simulink model "Australian14gen_inertia"  (R2017b)
settings: Solver=ode23tb  StartTime=0.0  StopTime=50  FixedStep=1e-3  RelTol=1e-3  AbsTol=1e-3  EnableMultiTasking=on
PreLoadFcn:
  | dataaustralian14gen
values from neighbouring files (symbols this model uses):
  alpha = -sys.follin.opt.alpha*1e8    [main_following.m]    (also in optimgains.mat = [-2447350365.29 -12566370614.4 -12566370614.4 -11730281347.7)
  bus_v = [ 101	15 ... (first row only)    [dataaustralian14gen.m]
  comp = [ 1	211	0	0 ... (first row only)    [dataaustralian14gen.m]
  dist = sys.follin.dist    [main_following.m]    (also in main_forming.m = sys.formin.dist)
  Exc = [ 101	0	 200	0.1	    13.25  2.5	 0	0       0       0       0       0 ... (first row only)    [dataaustralian14gen.m]
  FH = 13    [dataaustralian14gen.m]
  FI = 1    [dataaustralian14gen.m]
  FL = .1    (= 0.1)    [dataaustralian14gen.m]
  G_data = [ 101	333.3	15	3.6	0.14	1.1	0.65	0.25	8.5     0.25	0.05	0       0       0.25	0.2 	0 ... (first row only)    [dataaustralian14gen.m]
  KH = 120    [dataaustralian14gen.m]
  KI = 10    [dataaustralian14gen.m]
  KL = 10    [dataaustralian14gen.m]
  Kvsc = [-4.89904313526 -21.043852985 -7.4754770322 -20.8245159401 -7.65455531538 -20.65157337 -7.20128124012 -20.8334958357 -6.74777960012 -20.6206111903 -7.78863485578 -20.7555924998 ... (30 elements, 2x15)]    [optimgains.mat]
  line = [ 102	217	0.0084	0.0667	0.817	330	1 ... (first row only)    [dataaustralian14gen.m]
  load_mag = load_case4    [dataaustralian14gen.m]
  p = p_case4    [dataaustralian14gen.m]
  Pinit = zeros(15,1)    [dataaustralian14gen.m]
  PLL_Ki = 2/500    (= 0.004)    [dataaustralian14gen.m]
  PLL_Kp = 2/500    (= 0.004)    [dataaustralian14gen.m]
  PSSMODEL = 1    [dataaustralian14gen.m]
  trans = [ 1	101	102	15	330	333.3	12	12 ... (first row only)    [dataaustralian14gen.m]
undefined symbols (not defined in the file or in its folder): D1, Delta, sys, thetavsc0, Vbase
libraries: powerlib x388, Library x60, powerlib_meascontrol x15, sps_avr x10, powerlib_extras x4
(part 4 of 5)

== system Australian14gen_inertia/VI215_form ==
  Complex to Magnitude-Angle : ComplexToMagnitudeAngle
  Complex to Magnitude-Angle1 : ComplexToMagnitudeAngle
  Demux : Demux  Outputs=[3 3]
  Filter215 : Library/Filter  r=r_fil  l=l_fil  c=c_fil
  Gain : Gain  Gain=[1 0 0]  Multiplication=Matrix(K*u) (u vector)
  Gain1 : Gain  Gain=[1 0 0]  Multiplication=Matrix(K*u) (u vector)
  INV215 : Library/INV  fn=50  Ub=Vbase(4)  Pref=Pinit(4)  ang=thetavsc0(4)  K2=Kvsc(1,4)  K1=Kvsc(2,4)
  Load Flow Bus26 : powerlib/Measurements/Load Flow Bus  Commented=on  LConnTagsString=a  Phases=single  Connectors=on one side  ID=B215_vsw  Vbase=20e3  Vref=1  Vangle=0  VLF=1  VLFb=1  VLFc=1  angleLF=23.87  angleLFb=0  angleLFc=0
      settings: AttributesFormatString=%<ID>\n%<Vbase>V\n%<VLF>pu\n%<angleLF>deg.  SourceProductName=Simscape Power Systems
  Mux : Mux  Inputs=2
  Mux1 : Mux  Inputs=2
  Mux29 : Mux  Inputs=3
  Scope : Scope
  Scope1 : Scope  NumInputPorts=2
  Sum : Sum  Inputs=|+-
  fake_VSC_215 : powerlib/Electrical Sources/Three-Phase Source  Commented=on  InternalConnection=Yg  VoltagePhases=off  Voltage=(20000)*1  PhaseAngle=23.8703  Voltage_phases=[25e3 25e3 25e3]/sqrt(3)  PhaseAngles_phases=[0 -120 +120]  Frequency=50  NonIdealSource=off  SpecifyImpedance=off  Resistance=0  Inductance=0  ShortCircuitLevel=100e6  BaseVoltage=20e3  XRratio=7  BusType=PV  Pref=0  Qref=0  Prefabc=[10e3, 10e3, 10e3]  Qrefabc=[0, 0, 0]  Qmin=-inf  Qmax=inf
  u215 : Constant  Value=0
  A : PMIOPort  Port=1  Side=Left
  B : PMIOPort  Port=2  Side=Left
  C : PMIOPort  Port=3  Side=Left
  tag scope: P215=global, Q215=global, w215=global
  wires:
  u215/1 -> INV215/1
  INV215/3 -> Mux29/2
  INV215/2 -> Mux29/1
  Filter215/2 -> [Q215]
  INV215/1 -> [P215]
  INV215/4 -> Mux29/3
  Mux29/1 -> [w215]
  Filter215/1 -> INV215/2
  Mux/1 -> Scope1/1
  Sum/1 -> Scope/1
  Complex to Magnitude-Angle1/2 -> Mux1/2
  Gain/1 -> Complex to Magnitude-Angle/1
  Complex to Magnitude-Angle/1 -> Mux/1
  Demux/2 -> Gain1/1, Sum/2
  Filter215/3 -> Demux/1
  Demux/1 -> Gain/1, Sum/1
  Complex to Magnitude-Angle/2 -> Mux1/1
  Gain1/1 -> Complex to Magnitude-Angle1/1
  Mux1/1 -> Scope1/2
  Complex to Magnitude-Angle1/1 -> Mux/2
  connections:
  Filter215/LConn1 -- INV215/LConn1 -- Load Flow Bus26/LConn1 -- fake_VSC_215/RConn1
  Filter215/LConn2 -- INV215/LConn2 -- fake_VSC_215/RConn2
  Filter215/LConn3 -- INV215/LConn3 -- fake_VSC_215/RConn3
  C/RConn1 -- Filter215/RConn3
  Filter215/RConn2 -- B/RConn1
  A/RConn1 -- Filter215/RConn1

== system Australian14gen_inertia/VI216 ==
  Constant : Constant  Value=0
  Gain : Gain  Gain=-1
  Gain1 : Gain  Gain=[0 1]  Multiplication=Matrix(K*u) (u vector)
  Mux : Mux  Inputs=2
  Mux1 : Mux  Inputs=3
  PLL : Library/PLL  Kp=PLL_Kp  Ki=PLL_Ki  tau=PLL_tau  theta0=14.521  omega0=0
  "Power (3ph, Phasor)" : powerlib_meascontrol/Measurements/Power (3ph, Phasor)
      settings: SourceProductName=Simscape Power Systems  SourceProductBaseCode=PS
  Three-Phase V-I Measurement : powerlib/Measurements/Three-Phase V-I Measurement  VoltageMeasurement=phase-to-ground  SetLabelV=off  LabelV=Vabc  Vpu=off  VpuLL=off  CurrentMeasurement=yes  SetLabelI=off  LabelI=Iabc  Ipu=off  Pbase=100e6  Vbase=500e3  OutputType=Complex  PhasorSimulation=on  PSBequivalent=0
  dP102_vi : Library/dP102_vi  d=alpha(5)  m=alpha(20)
  virtin : powerlib/Elements/Three-Phase Dynamic Load  NominalVoltage=[20e3 50 ]  ActiveReactivePowers=[0 0]  PositiveSequence=[1.0263 14.521]  ExternalControl=on  NpNq="[0  0]"  TimeConstants="[0  0  0  0]"  MinimumVoltage=0.01  Tfilter=1e-1  LoadFlowParameters=[4 50000000 0 0 25000000]
      settings: SourceProductName=Simscape Power Systems  SourceProductBaseCode=PS
  A : PMIOPort  Port=1  Side=Right
  B : PMIOPort  Port=2  Side=Right
  C : PMIOPort  Port=3  Side=Right
  tag scope: P216=global, Q216=global, w216=global
  wires:
  Mux/1 -> Gain/1
  Gain/1 -> virtin/1
  Constant/1 -> Mux/2
  dP102_vi/1 -> Mux/1
  [Vabc_B216_vi] -> PLL/1
  PLL/1 -> Mux1/1, dP102_vi/1
  Mux1/1 -> [w216]
  PLL/2 -> Mux1/2, dP102_vi/2
  "Power (3ph, Phasor)"/1 -> [P216]
  Three-Phase V-I Measurement/1 -> "Power (3ph, Phasor)"/1
  "Power (3ph, Phasor)"/2 -> [Q216]
  Three-Phase V-I Measurement/2 -> "Power (3ph, Phasor)"/2
  PLL/3 -> Gain1/1
  Gain1/1 -> Mux1/3
  connections:
  C/RConn1 -- Three-Phase V-I Measurement/RConn3
  B/RConn1 -- Three-Phase V-I Measurement/RConn2
  A/RConn1 -- Three-Phase V-I Measurement/RConn1
  virtin/LConn3 -- Three-Phase V-I Measurement/LConn3
  virtin/LConn2 -- Three-Phase V-I Measurement/LConn2
  virtin/LConn1 -- Three-Phase V-I Measurement/LConn1

== system Australian14gen_inertia/VI216_form ==
  Complex to Magnitude-Angle : ComplexToMagnitudeAngle
  Complex to Magnitude-Angle1 : ComplexToMagnitudeAngle
  Demux : Demux  Outputs=[3 3]
  Filter216 : Library/Filter  r=r_fil  l=l_fil  c=c_fil
  Gain : Gain  Gain=[1 0 0]  Multiplication=Matrix(K*u) (u vector)
  Gain1 : Gain  Gain=[1 0 0]  Multiplication=Matrix(K*u) (u vector)
  INV216 : Library/INV  fn=50  Ub=Vbase(5)  Pref=Pinit(5)  ang=thetavsc0(5)  K2=Kvsc(1,5)  K1=Kvsc(2,5)
  Load Flow Bus25 : powerlib/Measurements/Load Flow Bus  Commented=on  LConnTagsString=a  Phases=single  Connectors=on one side  ID=B216_vsw  Vbase=20e3  Vref=1  Vangle=0  VLF=1  VLFb=1  VLFc=1  angleLF=14.02  angleLFb=0  angleLFc=0
      settings: AttributesFormatString=%<ID>\n%<Vbase>V\n%<VLF>pu\n%<angleLF>deg.  SourceProductName=Simscape Power Systems
  Mux : Mux  Inputs=2
  Mux1 : Mux  Inputs=2
  Mux23 : Mux  Inputs=3
  Scope : Scope
  Scope1 : Scope  NumInputPorts=2
  Sum : Sum  Inputs=|+-
  fake_VSC_216 : powerlib/Electrical Sources/Three-Phase Source  Commented=on  InternalConnection=Yg  VoltagePhases=off  Voltage=(20000)*1  PhaseAngle=14.0249  Voltage_phases=[25e3 25e3 25e3]/sqrt(3)  PhaseAngles_phases=[0 -120 +120]  Frequency=50  NonIdealSource=off  SpecifyImpedance=off  Resistance=0  Inductance=0  ShortCircuitLevel=100e6  BaseVoltage=20e3  XRratio=7  BusType=PV  Pref=0  Qref=0  Prefabc=[10e3, 10e3, 10e3]  Qrefabc=[0, 0, 0]  Qmin=-inf  Qmax=inf
  u216 : Constant  Value=0
  A : PMIOPort  Port=1  Side=Left
  B : PMIOPort  Port=2  Side=Left
  C : PMIOPort  Port=3  Side=Left
  tag scope: P216=global, Q216=global, w216=global
  wires:
  INV216/3 -> Mux23/2
  Filter216/1 -> INV216/2
  u216/1 -> INV216/1
  INV216/4 -> Mux23/3
  Mux23/1 -> [w216]
  INV216/1 -> [P216]
  INV216/2 -> Mux23/1
  Filter216/2 -> [Q216]
  Mux/1 -> Scope1/1
  Sum/1 -> Scope/1
  Complex to Magnitude-Angle1/2 -> Mux1/2
  Gain/1 -> Complex to Magnitude-Angle/1
  Complex to Magnitude-Angle/1 -> Mux/1
  Demux/2 -> Gain1/1, Sum/2
  Filter216/3 -> Demux/1
  Demux/1 -> Gain/1, Sum/1
  Complex to Magnitude-Angle/2 -> Mux1/1
  Gain1/1 -> Complex to Magnitude-Angle1/1
  Mux1/1 -> Scope1/2
  Complex to Magnitude-Angle1/1 -> Mux/2
  connections:
  INV216/LConn3 -- Filter216/LConn3 -- fake_VSC_216/RConn3
  INV216/LConn2 -- Filter216/LConn2 -- fake_VSC_216/RConn2
  Load Flow Bus25/LConn1 -- Filter216/LConn1 -- fake_VSC_216/RConn1 -- INV216/LConn1
  Filter216/RConn1 -- A/RConn1
  Filter216/RConn2 -- B/RConn1
  Filter216/RConn3 -- C/RConn1

== system Australian14gen_inertia/VI308 ==
  Constant : Constant  Value=0
  Gain : Gain  Gain=-1
  Gain1 : Gain  Gain=[0 1]  Multiplication=Matrix(K*u) (u vector)
  Mux : Mux  Inputs=2
  Mux1 : Mux  Inputs=3
  PLL : Library/PLL  Kp=PLL_Kp  Ki=PLL_Ki  tau=PLL_tau  theta0=-6.09646  omega0=0
  "Power (3ph, Phasor)" : powerlib_meascontrol/Measurements/Power (3ph, Phasor)
      settings: SourceProductName=Simscape Power Systems  SourceProductBaseCode=PS
  Three-Phase V-I Measurement : powerlib/Measurements/Three-Phase V-I Measurement  VoltageMeasurement=phase-to-ground  SetLabelV=off  LabelV=Vabc  Vpu=off  VpuLL=off  CurrentMeasurement=yes  SetLabelI=off  LabelI=Iabc  Ipu=off  Pbase=100e6  Vbase=500e3  OutputType=Complex  PhasorSimulation=on  PSBequivalent=0
  dP102_vi : Library/dP102_vi  d=alpha(6)  m=alpha(21)
  virtin : powerlib/Elements/Three-Phase Dynamic Load  NominalVoltage=[ 20e3 50 ]  ActiveReactivePowers=[0 0]  PositiveSequence=[1.0559 -6.09646]  ExternalControl=on  NpNq="[0  0]"  TimeConstants="[0  0  0  0]"  MinimumVoltage=0.01  Tfilter=1e-1  LoadFlowParameters=[4 50000000 0 0 25000000]
      settings: SourceProductName=Simscape Power Systems  SourceProductBaseCode=PS
  A : PMIOPort  Port=1  Side=Right
  B : PMIOPort  Port=2  Side=Right
  C : PMIOPort  Port=3  Side=Right
  tag scope: P308=global, Q308=global, w308=global
  wires:
  Mux/1 -> Gain/1
  Gain/1 -> virtin/1
  Constant/1 -> Mux/2
  dP102_vi/1 -> Mux/1
  [Vabc_B308_vi] -> PLL/1
  PLL/1 -> Mux1/1, dP102_vi/1
  Mux1/1 -> [w308]
  PLL/2 -> dP102_vi/2, Mux1/2
  "Power (3ph, Phasor)"/1 -> [P308]
  Three-Phase V-I Measurement/1 -> "Power (3ph, Phasor)"/1
  "Power (3ph, Phasor)"/2 -> [Q308]
  Three-Phase V-I Measurement/2 -> "Power (3ph, Phasor)"/2
  PLL/3 -> Gain1/1
  Gain1/1 -> Mux1/3
  connections:
  virtin/LConn1 -- Three-Phase V-I Measurement/LConn1
  C/RConn1 -- Three-Phase V-I Measurement/RConn3
  virtin/LConn3 -- Three-Phase V-I Measurement/LConn3
  B/RConn1 -- Three-Phase V-I Measurement/RConn2
  virtin/LConn2 -- Three-Phase V-I Measurement/LConn2
  A/RConn1 -- Three-Phase V-I Measurement/RConn1

== system Australian14gen_inertia/VI308_form ==
  Complex to Magnitude-Angle : ComplexToMagnitudeAngle
  Complex to Magnitude-Angle1 : ComplexToMagnitudeAngle
  Demux : Demux  Outputs=[3 3]
  Filter308 : Library/Filter  r=r_fil  l=l_fil  c=c_fil
  Gain : Gain  Gain=[1 0 0]  Multiplication=Matrix(K*u) (u vector)
  Gain1 : Gain  Gain=[1 0 0]  Multiplication=Matrix(K*u) (u vector)
  INV308 : Library/INV  fn=50  Ub=Vbase(6)  Pref=Pinit(6)  ang=thetavsc0(6)  K2=Kvsc(1,6)  K1=Kvsc(2,6)
  Load Flow Bus20 : powerlib/Measurements/Load Flow Bus  Commented=on  LConnTagsString=a  Phases=single  Connectors=on one side  ID=B308_vsw  Vbase=20e3  Vref=1  Vangle=0  VLF=1  VLFb=1  VLFc=1  angleLF=-6.338  angleLFb=0  angleLFc=0
      settings: AttributesFormatString=%<ID>\n%<Vbase>V\n%<VLF>pu\n%<angleLF>deg.  SourceProductName=Simscape Power Systems
  Mux : Mux  Inputs=2
  Mux1 : Mux  Inputs=2
  Mux19 : Mux  Inputs=3
  Scope : Scope
  Scope1 : Scope  NumInputPorts=2
  Sum : Sum  Inputs=|+-
  fake_VSC_308 : powerlib/Electrical Sources/Three-Phase Source  Commented=on  InternalConnection=Yg  VoltagePhases=off  Voltage=(20000)*1  PhaseAngle=-6.3379  Voltage_phases=[25e3 25e3 25e3]/sqrt(3)  PhaseAngles_phases=[0 -120 +120]  Frequency=50  NonIdealSource=off  SpecifyImpedance=off  Resistance=0  Inductance=0  ShortCircuitLevel=100e6  BaseVoltage=20e3  XRratio=7  BusType=PV  Pref=0  Qref=0  Prefabc=[10e3, 10e3, 10e3]  Qrefabc=[0, 0, 0]  Qmin=-inf  Qmax=inf
  u308 : Constant  Value=0
  A : PMIOPort  Port=1  Side=Left
  B : PMIOPort  Port=2  Side=Left
  C : PMIOPort  Port=3  Side=Left
  tag scope: P308=global, Q308=global, w308=global
  wires:
  INV308/4 -> Mux19/3
  Mux19/1 -> [w308]
  u308/1 -> INV308/1
  INV308/2 -> Mux19/1
  INV308/3 -> Mux19/2
  INV308/1 -> [P308]
  Filter308/1 -> INV308/2
  Filter308/2 -> [Q308]
  Mux/1 -> Scope1/1
  Sum/1 -> Scope/1
  Complex to Magnitude-Angle1/2 -> Mux1/2
  Gain/1 -> Complex to Magnitude-Angle/1
  Complex to Magnitude-Angle/1 -> Mux/1
  Demux/2 -> Gain1/1, Sum/2
  Filter308/3 -> Demux/1
  Demux/1 -> Gain/1, Sum/1
  Complex to Magnitude-Angle/2 -> Mux1/1
  Gain1/1 -> Complex to Magnitude-Angle1/1
  Mux1/1 -> Scope1/2
  Complex to Magnitude-Angle1/1 -> Mux/2
  connections:
  INV308/LConn3 -- Load Flow Bus20/LConn1 -- Filter308/LConn3 -- fake_VSC_308/RConn3
  INV308/LConn1 -- fake_VSC_308/RConn1 -- Filter308/LConn1
  INV308/LConn2 -- fake_VSC_308/RConn2 -- Filter308/LConn2
  B/RConn1 -- Filter308/RConn2
  C/RConn1 -- Filter308/RConn3
  A/RConn1 -- Filter308/RConn1

== system Australian14gen_inertia/VI309 ==
  Constant : Constant  Value=0
  Gain : Gain  Gain=-1
  Gain1 : Gain  Gain=[0 1]  Multiplication=Matrix(K*u) (u vector)
  Mux : Mux  Inputs=2
  Mux1 : Mux  Inputs=3
  PLL : Library/PLL  Kp=PLL_Kp  Ki=PLL_Ki  tau=PLL_tau  theta0=126.6523  omega0=0
  "Power (3ph, Phasor)" : powerlib_meascontrol/Measurements/Power (3ph, Phasor)
      settings: SourceProductName=Simscape Power Systems  SourceProductBaseCode=PS
  Three-Phase V-I Measurement : powerlib/Measurements/Three-Phase V-I Measurement  VoltageMeasurement=phase-to-ground  SetLabelV=off  LabelV=Vabc  Vpu=off  VpuLL=off  CurrentMeasurement=yes  SetLabelI=off  LabelI=Iabc  Ipu=off  Pbase=100e6  Vbase=500e3  OutputType=Complex  PhasorSimulation=on  PSBequivalent=0
  dP102_vi : Library/dP102_vi  d=alpha(7)  m=alpha(22)
  virtin : powerlib/Elements/Three-Phase Dynamic Load  NominalVoltage=[ 15e3 50 ]  ActiveReactivePowers=[0 0]  PositiveSequence=[1.04736 5.11816]  ExternalControl=on  NpNq="[0  0]"  TimeConstants="[0  0  0  0]"  MinimumVoltage=0.01  Tfilter=1e-1  LoadFlowParameters=[4 50000000 0 0 25000000]
      settings: SourceProductName=Simscape Power Systems  SourceProductBaseCode=PS
  A : PMIOPort  Port=1  Side=Right
  B : PMIOPort  Port=2  Side=Right
  C : PMIOPort  Port=3  Side=Right
  tag scope: P309=global, Q309=global, w309=global
  wires:
  Mux/1 -> Gain/1
  Gain/1 -> virtin/1
  Constant/1 -> Mux/2
  dP102_vi/1 -> Mux/1
  [Vabc_B309_vi] -> PLL/1
  PLL/1 -> Mux1/1, dP102_vi/1
  Mux1/1 -> [w309]
  PLL/2 -> Mux1/2, dP102_vi/2
  "Power (3ph, Phasor)"/1 -> [P309]
  Three-Phase V-I Measurement/1 -> "Power (3ph, Phasor)"/1
  "Power (3ph, Phasor)"/2 -> [Q309]
  Three-Phase V-I Measurement/2 -> "Power (3ph, Phasor)"/2
  PLL/3 -> Gain1/1
  Gain1/1 -> Mux1/3
  connections:
  virtin/LConn1 -- Three-Phase V-I Measurement/LConn1
  C/RConn1 -- Three-Phase V-I Measurement/RConn3
  virtin/LConn3 -- Three-Phase V-I Measurement/LConn3
  B/RConn1 -- Three-Phase V-I Measurement/RConn2
  virtin/LConn2 -- Three-Phase V-I Measurement/LConn2
  A/RConn1 -- Three-Phase V-I Measurement/RConn1

== system Australian14gen_inertia/VI309_form ==
  Complex to Magnitude-Angle : ComplexToMagnitudeAngle
  Complex to Magnitude-Angle1 : ComplexToMagnitudeAngle
  Demux : Demux  Outputs=[3 3]
  Filter309 : Library/Filter  r=r_fil  l=l_fil  c=c_fil
  Gain : Gain  Gain=[1 0 0]  Multiplication=Matrix(K*u) (u vector)
  Gain1 : Gain  Gain=[1 0 0]  Multiplication=Matrix(K*u) (u vector)
  INV309 : Library/INV  fn=50  Ub=Vbase(7)  Pref=Pinit(7)  ang=thetavsc0(7)  K2=Kvsc(1,7)  K1=Kvsc(2,7)
  Load Flow Bus23 : powerlib/Measurements/Load Flow Bus  Commented=on  LConnTagsString=a  Phases=single  Connectors=on one side  ID=B309_vsw  Vbase=15e3  Vref=1  Vangle=0  VLF=1  VLFb=1  VLFc=1  angleLF=4.793  angleLFb=0  angleLFc=0
      settings: AttributesFormatString=%<ID>\n%<Vbase>V\n%<VLF>pu\n%<angleLF>deg.  SourceProductName=Simscape Power Systems
  Mux : Mux  Inputs=2
  Mux1 : Mux  Inputs=2
  Mux28 : Mux  Inputs=3
  Scope : Scope
  Scope1 : Scope  NumInputPorts=2
  Sum : Sum  Inputs=|+-
  fake_VSC_309 : powerlib/Electrical Sources/Three-Phase Source  Commented=on  InternalConnection=Yg  VoltagePhases=off  Voltage=(15000)*1  PhaseAngle=4.7928  Voltage_phases=[25e3 25e3 25e3]/sqrt(3)  PhaseAngles_phases=[0 -120 +120]  Frequency=50  NonIdealSource=off  SpecifyImpedance=off  Resistance=0  Inductance=0  ShortCircuitLevel=100e6  BaseVoltage=20e3  XRratio=7  BusType=PV  Pref=0  Qref=0  Prefabc=[10e3, 10e3, 10e3]  Qrefabc=[0, 0, 0]  Qmin=-inf  Qmax=inf
  u309 : Constant  Value=0
  A : PMIOPort  Port=1  Side=Right
  B : PMIOPort  Port=2  Side=Right
  C : PMIOPort  Port=3  Side=Right
  tag scope: P309=global, Q309=global, w309=global
  wires:
  INV309/1 -> [P309]
  Filter309/1 -> INV309/2
  INV309/3 -> Mux28/2
  Mux28/1 -> [w309]
  INV309/2 -> Mux28/1
  Filter309/2 -> [Q309]
  u309/1 -> INV309/1
  INV309/4 -> Mux28/3
  Mux/1 -> Scope1/1
  Sum/1 -> Scope/1
  Complex to Magnitude-Angle1/2 -> Mux1/2
  Gain/1 -> Complex to Magnitude-Angle/1
  Complex to Magnitude-Angle/1 -> Mux/1
  Demux/2 -> Gain1/1, Sum/2
  Filter309/3 -> Demux/1
  Demux/1 -> Gain/1, Sum/1
  Complex to Magnitude-Angle/2 -> Mux1/1
  Gain1/1 -> Complex to Magnitude-Angle1/1
  Mux1/1 -> Scope1/2
  Complex to Magnitude-Angle1/1 -> Mux/2
  connections:
  INV309/LConn3 -- fake_VSC_309/RConn3 -- Filter309/LConn3
  INV309/LConn1 -- Load Flow Bus23/LConn1 -- Filter309/LConn1 -- fake_VSC_309/RConn1
  INV309/LConn2 -- fake_VSC_309/RConn2 -- Filter309/LConn2
  A/RConn1 -- Filter309/RConn1
  B/RConn1 -- Filter309/RConn2
  C/RConn1 -- Filter309/RConn3

== system Australian14gen_inertia/VI312 ==
  Constant : Constant  Value=0
  Gain : Gain  Gain=-1
  Gain1 : Gain  Gain=[0 1]  Multiplication=Matrix(K*u) (u vector)
  Mux : Mux  Inputs=2
  Mux1 : Mux  Inputs=3
  PLL : Library/PLL  Kp=PLL_Kp  Ki=PLL_Ki  tau=PLL_tau  theta0=3.98868  omega0=0
  "Power (3ph, Phasor)" : powerlib_meascontrol/Measurements/Power (3ph, Phasor)
      settings: SourceProductName=Simscape Power Systems  SourceProductBaseCode=PS
  Three-Phase V-I Measurement : powerlib/Measurements/Three-Phase V-I Measurement  VoltageMeasurement=phase-to-ground  SetLabelV=off  LabelV=Vabc  Vpu=off  VpuLL=off  CurrentMeasurement=yes  SetLabelI=off  LabelI=Iabc  Ipu=off  Pbase=100e6  Vbase=500e3  OutputType=Complex  PhasorSimulation=on  PSBequivalent=0
  dP102_vi : Library/dP102_vi  d=alpha(8)  m=alpha(23)
  virtin : powerlib/Elements/Three-Phase Dynamic Load  NominalVoltage=[ 20e3 50 ]  ActiveReactivePowers=[0 0]  PositiveSequence=[0.998867 3.98868]  ExternalControl=on  NpNq="[0  0]"  TimeConstants="[0  0  0  0]"  MinimumVoltage=0.01  Tfilter=1e-1  LoadFlowParameters=[4 50000000 0 0 25000000]
      settings: SourceProductName=Simscape Power Systems  SourceProductBaseCode=PS
  A : PMIOPort  Port=1  Side=Right
  B : PMIOPort  Port=2  Side=Right
  C : PMIOPort  Port=3  Side=Right
  tag scope: P312=global, Q312=global, w312=global
  wires:
  Mux/1 -> Gain/1
  Gain/1 -> virtin/1
  Constant/1 -> Mux/2
  dP102_vi/1 -> Mux/1
  [Vabc_B312_vi] -> PLL/1
  PLL/1 -> Mux1/1, dP102_vi/1
  Mux1/1 -> [w312]
  PLL/2 -> Mux1/2, dP102_vi/2
  "Power (3ph, Phasor)"/1 -> [P312]
  Three-Phase V-I Measurement/1 -> "Power (3ph, Phasor)"/1
  "Power (3ph, Phasor)"/2 -> [Q312]
  Three-Phase V-I Measurement/2 -> "Power (3ph, Phasor)"/2
  PLL/3 -> Gain1/1
  Gain1/1 -> Mux1/3
  connections:
  virtin/LConn1 -- Three-Phase V-I Measurement/LConn1
  C/RConn1 -- Three-Phase V-I Measurement/RConn3
  virtin/LConn3 -- Three-Phase V-I Measurement/LConn3
  B/RConn1 -- Three-Phase V-I Measurement/RConn2
  virtin/LConn2 -- Three-Phase V-I Measurement/LConn2
  A/RConn1 -- Three-Phase V-I Measurement/RConn1

== system Australian14gen_inertia/VI312_form ==
  Complex to Magnitude-Angle : ComplexToMagnitudeAngle
  Complex to Magnitude-Angle1 : ComplexToMagnitudeAngle
  Demux : Demux  Outputs=[3 3]
  Filter312 : Library/Filter  r=r_fil  l=l_fil  c=c_fil
  Gain : Gain  Gain=[1 0 0]  Multiplication=Matrix(K*u) (u vector)
  Gain1 : Gain  Gain=[1 0 0]  Multiplication=Matrix(K*u) (u vector)
  INV312 : Library/INV  fn=50  Ub=Vbase(8)  Pref=Pinit(8)  ang=thetavsc0(8)  K2=Kvsc(1,8)  K1=Kvsc(2,8)
  Load Flow Bus22 : powerlib/Measurements/Load Flow Bus  Commented=on  LConnTagsString=a  Phases=single  Connectors=on one side  ID=B312_vsw  Vbase=20e3  Vref=1  Vangle=0  VLF=1  VLFb=1  VLFc=1  angleLF=3.684  angleLFb=0  angleLFc=0
      settings: AttributesFormatString=%<ID>\n%<Vbase>V\n%<VLF>pu\n%<angleLF>deg.  SourceProductName=Simscape Power Systems
  Mux : Mux  Inputs=2
  Mux1 : Mux  Inputs=2
  Mux17 : Mux  Inputs=3
  Scope : Scope
  Scope1 : Scope  NumInputPorts=2
  Sum : Sum  Inputs=|+-
  fake_VSC_312 : powerlib/Electrical Sources/Three-Phase Source  Commented=on  InternalConnection=Yg  VoltagePhases=off  Voltage=(20000)*1  PhaseAngle=3.6837  Voltage_phases=[25e3 25e3 25e3]/sqrt(3)  PhaseAngles_phases=[0 -120 +120]  Frequency=50  NonIdealSource=off  SpecifyImpedance=off  Resistance=0  Inductance=0  ShortCircuitLevel=100e6  BaseVoltage=20e3  XRratio=7  BusType=PV  Pref=0  Qref=0  Prefabc=[10e3, 10e3, 10e3]  Qrefabc=[0, 0, 0]  Qmin=-inf  Qmax=inf
  u312 : Constant  Value=0
  A : PMIOPort  Port=1  Side=Left
  B : PMIOPort  Port=2  Side=Left
  C : PMIOPort  Port=3  Side=Left
  tag scope: P312=global, Q312=global, w312=global
  wires:
  Filter312/2 -> [Q312]
  INV312/1 -> [P312]
  Filter312/1 -> INV312/2
  INV312/3 -> Mux17/2
  u312/1 -> INV312/1
  INV312/2 -> Mux17/1
  INV312/4 -> Mux17/3
  Mux17/1 -> [w312]
  Mux/1 -> Scope1/1
  Sum/1 -> Scope/1
  Complex to Magnitude-Angle1/2 -> Mux1/2
  Gain/1 -> Complex to Magnitude-Angle/1
  Complex to Magnitude-Angle/1 -> Mux/1
  Demux/2 -> Gain1/1, Sum/2
  Filter312/3 -> Demux/1
  Demux/1 -> Gain/1, Sum/1
  Complex to Magnitude-Angle/2 -> Mux1/1
  Gain1/1 -> Complex to Magnitude-Angle1/1
  Mux1/1 -> Scope1/2
  Complex to Magnitude-Angle1/1 -> Mux/2
  connections:
  INV312/LConn3 -- fake_VSC_312/RConn3 -- Filter312/LConn3
  INV312/LConn2 -- fake_VSC_312/RConn2 -- Filter312/LConn2
  INV312/LConn1 -- Load Flow Bus22/LConn1 -- fake_VSC_312/RConn1 -- Filter312/LConn1
  C/RConn1 -- Filter312/RConn3
  B/RConn1 -- Filter312/RConn2
  A/RConn1 -- Filter312/RConn1

== system Australian14gen_inertia/VI314 ==
  Constant : Constant  Value=0
  Gain : Gain  Gain=-1
  Gain1 : Gain  Gain=[0 1]  Multiplication=Matrix(K*u) (u vector)
  Mux : Mux  Inputs=2
  Mux1 : Mux  Inputs=3
  PLL : Library/PLL  Kp=PLL_Kp  Ki=PLL_Ki  tau=PLL_tau  theta0=-0.807945  omega0=0
  "Power (3ph, Phasor)" : powerlib_meascontrol/Measurements/Power (3ph, Phasor)
      settings: SourceProductName=Simscape Power Systems  SourceProductBaseCode=PS
  Three-Phase V-I Measurement : powerlib/Measurements/Three-Phase V-I Measurement  VoltageMeasurement=phase-to-ground  SetLabelV=off  LabelV=Vabc  Vpu=off  VpuLL=off  CurrentMeasurement=yes  SetLabelI=off  LabelI=Iabc  Ipu=off  Pbase=100e6  Vbase=500e3  OutputType=Complex  PhasorSimulation=on  PSBequivalent=0
  dP102_vi : Library/dP102_vi  d=alpha(9)  m=alpha(24)
  virtin : powerlib/Elements/Three-Phase Dynamic Load  NominalVoltage=[ 20e3 50 ]  ActiveReactivePowers=[0 0]  PositiveSequence=[0.999559 -0.807945]  ExternalControl=on  NpNq="[0  0]"  TimeConstants="[0  0  0  0]"  MinimumVoltage=0.01  Tfilter=1e-1  LoadFlowParameters=[4 50000000 0 0 25000000]
      settings: SourceProductName=Simscape Power Systems  SourceProductBaseCode=PS
  A : PMIOPort  Port=1  Side=Right
  B : PMIOPort  Port=2  Side=Right
  C : PMIOPort  Port=3  Side=Right
  tag scope: P314=global, Q314=global, w314=global
  wires:
  Mux/1 -> Gain/1
  Gain/1 -> virtin/1
  Constant/1 -> Mux/2
  dP102_vi/1 -> Mux/1
  [Vabc_B314_vi] -> PLL/1
  PLL/1 -> Mux1/1, dP102_vi/1
  Mux1/1 -> [w314]
  PLL/2 -> Mux1/2, dP102_vi/2
  "Power (3ph, Phasor)"/1 -> [P314]
  Three-Phase V-I Measurement/1 -> "Power (3ph, Phasor)"/1
  "Power (3ph, Phasor)"/2 -> [Q314]
  Three-Phase V-I Measurement/2 -> "Power (3ph, Phasor)"/2
  PLL/3 -> Gain1/1
  Gain1/1 -> Mux1/3
  connections:
  virtin/LConn1 -- Three-Phase V-I Measurement/LConn1
  C/RConn1 -- Three-Phase V-I Measurement/RConn3
  virtin/LConn3 -- Three-Phase V-I Measurement/LConn3
  B/RConn1 -- Three-Phase V-I Measurement/RConn2
  virtin/LConn2 -- Three-Phase V-I Measurement/LConn2
  A/RConn1 -- Three-Phase V-I Measurement/RConn1

== system Australian14gen_inertia/VI314_form ==
  Complex to Magnitude-Angle : ComplexToMagnitudeAngle
  Complex to Magnitude-Angle1 : ComplexToMagnitudeAngle
  Demux : Demux  Outputs=[3 3]
  Filter314 : Library/Filter  r=r_fil  l=l_fil  c=c_fil
  Gain : Gain  Gain=[1 0 0]  Multiplication=Matrix(K*u) (u vector)
  Gain1 : Gain  Gain=[1 0 0]  Multiplication=Matrix(K*u) (u vector)
  INV314 : Library/INV  fn=50  Ub=Vbase(9)  Pref=Pinit(9)  ang=thetavsc0(9)  K2=Kvsc(1,9)  K1=Kvsc(2,9)
  Load Flow Bus21 : powerlib/Measurements/Load Flow Bus  Commented=on  LConnTagsString=a  Phases=single  Connectors=on one side  ID=B314_vsw  Vbase=20e3  Vref=1  Vangle=0  VLF=1  VLFb=1  VLFc=1  angleLF=-1.099  angleLFb=0  angleLFc=0
      settings: AttributesFormatString=%<ID>\n%<Vbase>V\n%<VLF>pu\n%<angleLF>deg.  SourceProductName=Simscape Power Systems
  Mux : Mux  Inputs=2
  Mux1 : Mux  Inputs=2
  Mux18 : Mux  Inputs=3
  Scope : Scope
  Scope1 : Scope  NumInputPorts=2
  Sum : Sum  Inputs=|+-
  fake_VSC_314 : powerlib/Electrical Sources/Three-Phase Source  Commented=on  InternalConnection=Yg  VoltagePhases=off  Voltage=(20000)*1  PhaseAngle=-1.0986  Voltage_phases=[25e3 25e3 25e3]/sqrt(3)  PhaseAngles_phases=[0 -120 +120]  Frequency=50  NonIdealSource=off  SpecifyImpedance=off  Resistance=0  Inductance=0  ShortCircuitLevel=100e6  BaseVoltage=20e3  XRratio=7  BusType=PV  Pref=0  Qref=0  Prefabc=[10e3, 10e3, 10e3]  Qrefabc=[0, 0, 0]  Qmin=-inf  Qmax=inf
  u314 : Constant  Value=0
  A : PMIOPort  Port=1  Side=Left
  B : PMIOPort  Port=2  Side=Left
  C : PMIOPort  Port=3  Side=Left
  tag scope: P314=global, Q314=global, w314=global
  wires:
  INV314/4 -> Mux18/3
  u314/1 -> INV314/1
  INV314/2 -> Mux18/1
  INV314/3 -> Mux18/2
  Filter314/2 -> [Q314]
  Mux18/1 -> [w314]
  Filter314/1 -> INV314/2
  INV314/1 -> [P314]
  Mux/1 -> Scope1/1
  Sum/1 -> Scope/1
  Complex to Magnitude-Angle1/2 -> Mux1/2
  Gain/1 -> Complex to Magnitude-Angle/1
  Complex to Magnitude-Angle/1 -> Mux/1
  Demux/2 -> Gain1/1, Sum/2
  Filter314/3 -> Demux/1
  Demux/1 -> Gain/1, Sum/1
  Complex to Magnitude-Angle/2 -> Mux1/1
  Gain1/1 -> Complex to Magnitude-Angle1/1
  Mux1/1 -> Scope1/2
  Complex to Magnitude-Angle1/1 -> Mux/2
  connections:
  INV314/LConn1 -- fake_VSC_314/RConn1 -- Filter314/LConn1
  INV314/LConn3 -- fake_VSC_314/RConn3 -- Load Flow Bus21/LConn1 -- Filter314/LConn3
  INV314/LConn2 -- fake_VSC_314/RConn2 -- Filter314/LConn2
  A/RConn1 -- Filter314/RConn1
  B/RConn1 -- Filter314/RConn2
  C/RConn1 -- Filter314/RConn3

== system Australian14gen_inertia/VI403 ==
  Constant : Constant  Value=0
  Gain : Gain  Gain=-1
  Gain1 : Gain  Gain=[0 1]  Multiplication=Matrix(K*u) (u vector)
  Mux : Mux  Inputs=2
  Mux1 : Mux  Inputs=3
  PLL : Library/PLL  Kp=PLL_Kp  Ki=PLL_Ki  tau=PLL_tau  theta0=29.6583  omega0=0
  "Power (3ph, Phasor)" : powerlib_meascontrol/Measurements/Power (3ph, Phasor)
      settings: SourceProductName=Simscape Power Systems  SourceProductBaseCode=PS
  Three-Phase V-I Measurement : powerlib/Measurements/Three-Phase V-I Measurement  VoltageMeasurement=phase-to-ground  SetLabelV=off  LabelV=Vabc  Vpu=off  VpuLL=off  CurrentMeasurement=yes  SetLabelI=off  LabelI=Iabc  Ipu=off  Pbase=100e6  Vbase=500e3  OutputType=Complex  PhasorSimulation=on  PSBequivalent=0
  dP102_vi : Library/dP102_vi  d=alpha(10)  m=alpha(25)
  virtin : powerlib/Elements/Three-Phase Dynamic Load  NominalVoltage=[ 20e3 50 ]  ActiveReactivePowers=[0 0]  PositiveSequence=[0.997203 20.5817]  ExternalControl=on  NpNq="[0  0]"  TimeConstants="[0  0  0  0]"  MinimumVoltage=0.01  Tfilter=1e-1  LoadFlowParameters=[4 50000000 0 0 25000000]
      settings: SourceProductName=Simscape Power Systems  SourceProductBaseCode=PS
  A : PMIOPort  Port=1  Side=Right
  B : PMIOPort  Port=2  Side=Right
  C : PMIOPort  Port=3  Side=Right
  tag scope: P403=global, Q403=global, w403=global
  wires:
  Mux/1 -> Gain/1
  Gain/1 -> virtin/1
  Constant/1 -> Mux/2
  dP102_vi/1 -> Mux/1
  [Vabc_B403] -> PLL/1
  PLL/1 -> Mux1/1, dP102_vi/1
  Mux1/1 -> [w403]
  PLL/2 -> Mux1/2, dP102_vi/2
  PLL/3 -> Gain1/1
  Three-Phase V-I Measurement/1 -> "Power (3ph, Phasor)"/1
  Three-Phase V-I Measurement/2 -> "Power (3ph, Phasor)"/2
  Gain1/1 -> Mux1/3
  "Power (3ph, Phasor)"/2 -> [Q403]
  "Power (3ph, Phasor)"/1 -> [P403]
  connections:
  B/RConn1 -- Three-Phase V-I Measurement/RConn2
  A/RConn1 -- Three-Phase V-I Measurement/RConn1
  C/RConn1 -- Three-Phase V-I Measurement/RConn3
  virtin/LConn1 -- Three-Phase V-I Measurement/LConn1
  virtin/LConn3 -- Three-Phase V-I Measurement/LConn3
  virtin/LConn2 -- Three-Phase V-I Measurement/LConn2

== system Australian14gen_inertia/VI403_form ==
  Complex to Magnitude-Angle : ComplexToMagnitudeAngle
  Complex to Magnitude-Angle1 : ComplexToMagnitudeAngle
  Demux : Demux  Outputs=[3 3]
  Filter403 : Library/Filter  r=r_fil  l=l_fil  c=c_fil
  Gain : Gain  Gain=[1 0 0]  Multiplication=Matrix(K*u) (u vector)
  Gain1 : Gain  Gain=[1 0 0]  Multiplication=Matrix(K*u) (u vector)
  INV403 : Library/INV  fn=50  Ub=Vbase(10)  Pref=Pinit(10)  ang=thetavsc0(10)  K2=Kvsc(1,10)  K1=Kvsc(2,10)
  Load Flow Bus1 : powerlib/Measurements/Load Flow Bus  Commented=on  LConnTagsString=a  Phases=single  Connectors=on one side  ID=B403_vsw  Vbase=20e3  Vref=1  Vangle=0  VLF=0.9972  VLFb=1  VLFc=1  angleLF=23.58  angleLFb=0  angleLFc=0
      settings: AttributesFormatString=%<ID>\n%<Vbase>V\n%<VLF>pu\n%<angleLF>deg.  SourceProductName=Simscape Power Systems
  Mux : Mux  Inputs=2
  Mux1 : Mux  Inputs=2
  Mux15 : Mux  Inputs=3
  Scope : Scope
  Scope1 : Scope  NumInputPorts=2
  Sum : Sum  Inputs=|+-
  fake_VSC_403 : powerlib/Electrical Sources/Three-Phase Source  Commented=on  InternalConnection=Yg  VoltagePhases=off  Voltage=(20000)*1  PhaseAngle=23.5812  Voltage_phases=[25e3 25e3 25e3]/sqrt(3)  PhaseAngles_phases=[0 -120 +120]  Frequency=50  NonIdealSource=off  SpecifyImpedance=off  Resistance=0  Inductance=0  ShortCircuitLevel=100e6  BaseVoltage=20e3  XRratio=7  BusType=PV  Pref=0  Qref=0  Prefabc=[10e3, 10e3, 10e3]  Qrefabc=[0, 0, 0]  Qmin=-inf  Qmax=inf
  u403 : Constant  Value=0
  A : PMIOPort  Port=1  Side=Right
  B : PMIOPort  Port=2  Side=Right
  C : PMIOPort  Port=3  Side=Right
  tag scope: P403=global, Q403=global, w403=global
  wires:
  INV403/1 -> [P403]
  Filter403/2 -> [Q403]
  Mux15/1 -> [w403]
  Filter403/1 -> INV403/2
  INV403/2 -> Mux15/1
  INV403/3 -> Mux15/2
  u403/1 -> INV403/1
  INV403/4 -> Mux15/3
  Filter403/3 -> Demux/1
  Demux/1 -> Gain/1, Sum/1
  Demux/2 -> Gain1/1, Sum/2
  Sum/1 -> Scope/1
  Gain/1 -> Complex to Magnitude-Angle/1
  Gain1/1 -> Complex to Magnitude-Angle1/1
  Mux/1 -> Scope1/1
  Complex to Magnitude-Angle/1 -> Mux/1
  Complex to Magnitude-Angle1/1 -> Mux/2
  Mux1/1 -> Scope1/2
  Complex to Magnitude-Angle/2 -> Mux1/1
  Complex to Magnitude-Angle1/2 -> Mux1/2
  connections:
  Load Flow Bus1/LConn1 -- fake_VSC_403/RConn3 -- Filter403/LConn3 -- INV403/LConn3
  Filter403/LConn1 -- INV403/LConn1 -- fake_VSC_403/RConn1
  Filter403/LConn2 -- INV403/LConn2 -- fake_VSC_403/RConn2
  Filter403/RConn1 -- A/RConn1
  C/RConn1 -- Filter403/RConn3
  Filter403/RConn2 -- B/RConn1

== system Australian14gen_inertia/VI405 ==
  Constant : Constant  Value=0
  Gain : Gain  Gain=-1
  Gain1 : Gain  Gain=[0 1]  Multiplication=Matrix(K*u) (u vector)
  Mux : Mux  Inputs=2
  Mux1 : Mux  Inputs=3
  PLL : Library/PLL  Kp=PLL_Kp  Ki=PLL_Ki  tau=PLL_tau  theta0=16.7314  omega0=0
  "Power (3ph, Phasor)" : powerlib_meascontrol/Measurements/Power (3ph, Phasor)
      settings: SourceProductName=Simscape Power Systems  SourceProductBaseCode=PS
  Three-Phase V-I Measurement : powerlib/Measurements/Three-Phase V-I Measurement  VoltageMeasurement=phase-to-ground  SetLabelV=off  LabelV=Vabc  Vpu=off  VpuLL=off  CurrentMeasurement=yes  SetLabelI=off  LabelI=Iabc  Ipu=off  Pbase=100e6  Vbase=500e3  OutputType=Complex  PhasorSimulation=on  PSBequivalent=0
  dP102_vi : Library/dP102_vi  d=alpha(11)  m=alpha(26)
  virtin : powerlib/Elements/Three-Phase Dynamic Load  NominalVoltage=[20e3 50 ]  ActiveReactivePowers=[0 0]  PositiveSequence=[1.00896 16.7314]  ExternalControl=on  NpNq="[0  0]"  TimeConstants="[0  0  0  0]"  MinimumVoltage=0.01  Tfilter=1e-1  LoadFlowParameters=[4 50000000 0 0 25000000]
      settings: SourceProductName=Simscape Power Systems  SourceProductBaseCode=PS
  A : PMIOPort  Port=1  Side=Right
  B : PMIOPort  Port=2  Side=Right
  C : PMIOPort  Port=3  Side=Right
  tag scope: P405=global, Q405=global, w405=global
  wires:
  Mux/1 -> Gain/1
  Gain/1 -> virtin/1
  Constant/1 -> Mux/2
  dP102_vi/1 -> Mux/1
  [Vabc_B405_vi] -> PLL/1
  PLL/1 -> Mux1/1, dP102_vi/1
  Mux1/1 -> [w405]
  PLL/2 -> Mux1/2, dP102_vi/2
  "Power (3ph, Phasor)"/1 -> [P405]
  Three-Phase V-I Measurement/1 -> "Power (3ph, Phasor)"/1
  Three-Phase V-I Measurement/2 -> "Power (3ph, Phasor)"/2
  "Power (3ph, Phasor)"/2 -> [Q405]
  PLL/3 -> Gain1/1
  Gain1/1 -> Mux1/3
  connections:
  B/RConn1 -- Three-Phase V-I Measurement/RConn2
  A/RConn1 -- Three-Phase V-I Measurement/RConn1
  C/RConn1 -- Three-Phase V-I Measurement/RConn3
  virtin/LConn1 -- Three-Phase V-I Measurement/LConn1
  virtin/LConn3 -- Three-Phase V-I Measurement/LConn3
  virtin/LConn2 -- Three-Phase V-I Measurement/LConn2

== system Australian14gen_inertia/VI405_form ==
  Complex to Magnitude-Angle : ComplexToMagnitudeAngle
  Complex to Magnitude-Angle1 : ComplexToMagnitudeAngle
  Demux : Demux  Outputs=[3 3]
  Filter405 : Library/Filter  r=r_fil  l=l_fil  c=c_fil
  Gain : Gain  Gain=[1 0 0]  Multiplication=Matrix(K*u) (u vector)
  Gain1 : Gain  Gain=[1 0 0]  Multiplication=Matrix(K*u) (u vector)
  INV405 : Library/INV  fn=50  Ub=Vbase(11)  Pref=Pinit(11)  ang=thetavsc0(11)  K2=Kvsc(1,11)  K1=Kvsc(2,11)
  Load Flow Bus29 : powerlib/Measurements/Load Flow Bus  Commented=on  LConnTagsString=a  Phases=single  Connectors=on one side  ID=B405_vsw  Vbase=20e3  Vref=1  Vangle=0  VLF=0.9972  VLFb=1  VLFc=1  angleLF=23.58  angleLFb=0  angleLFc=0
      settings: AttributesFormatString=%<ID>\n%<Vbase>V\n%<VLF>pu\n%<angleLF>deg.  SourceProductName=Simscape Power Systems
  Mux : Mux  Inputs=2
  Mux1 : Mux  Inputs=2
  Mux16 : Mux  Inputs=3
  Scope : Scope
  Scope1 : Scope  NumInputPorts=2
  Sum : Sum  Inputs=|+-
  fake_VSC_405 : powerlib/Electrical Sources/Three-Phase Source  Commented=on  InternalConnection=Yg  VoltagePhases=off  Voltage=(20000)*1  PhaseAngle=10.5944  Voltage_phases=[25e3 25e3 25e3]/sqrt(3)  PhaseAngles_phases=[0 -120 +120]  Frequency=50  NonIdealSource=off  SpecifyImpedance=off  Resistance=0  Inductance=0  ShortCircuitLevel=100e6  BaseVoltage=20e3  XRratio=7  BusType=PV  Pref=0  Qref=0  Prefabc=[10e3, 10e3, 10e3]  Qrefabc=[0, 0, 0]  Qmin=-inf  Qmax=inf
  u405 : Constant  Value=0
  A : PMIOPort  Port=1  Side=Right
  B : PMIOPort  Port=2  Side=Right
  C : PMIOPort  Port=3  Side=Right
  tag scope: P405=global, Q405=global, w405=global
  wires:
  INV405/4 -> Mux16/3
  Filter405/2 -> [Q405]
  INV405/1 -> [P405]
  Mux16/1 -> [w405]
  INV405/2 -> Mux16/1
  INV405/3 -> Mux16/2
  u405/1 -> INV405/1
  Filter405/1 -> INV405/2
  Demux/1 -> Gain/1, Sum/1
  Gain/1 -> Complex to Magnitude-Angle/1
  Demux/2 -> Gain1/1, Sum/2
  Complex to Magnitude-Angle1/1 -> Mux/2
  Sum/1 -> Scope/1
  Mux/1 -> Scope1/1
  Complex to Magnitude-Angle/2 -> Mux1/1
  Mux1/1 -> Scope1/2
  Gain1/1 -> Complex to Magnitude-Angle1/1
  Filter405/3 -> Demux/1
  Complex to Magnitude-Angle1/2 -> Mux1/2
  Complex to Magnitude-Angle/1 -> Mux/1
  connections:
  INV405/LConn3 -- Load Flow Bus29/LConn1 -- Filter405/LConn3 -- fake_VSC_405/RConn3
  INV405/LConn2 -- fake_VSC_405/RConn2 -- Filter405/LConn2
  INV405/LConn1 -- fake_VSC_405/RConn1 -- Filter405/LConn1
  A/RConn1 -- Filter405/RConn1
  B/RConn1 -- Filter405/RConn2
  C/RConn1 -- Filter405/RConn3

== system Australian14gen_inertia/VI410 ==
  Constant : Constant  Value=0
  Gain : Gain  Gain=-1
  Gain1 : Gain  Gain=[0 1]  Multiplication=Matrix(K*u) (u vector)
  Mux : Mux  Inputs=2
  Mux1 : Mux  Inputs=3
  PLL : Library/PLL  Kp=PLL_Kp  Ki=PLL_Ki  tau=PLL_tau  theta0=8.97655  omega0=0
  "Power (3ph, Phasor)" : powerlib_meascontrol/Measurements/Power (3ph, Phasor)
      settings: SourceProductName=Simscape Power Systems  SourceProductBaseCode=PS
  Three-Phase V-I Measurement : powerlib/Measurements/Three-Phase V-I Measurement  VoltageMeasurement=phase-to-ground  SetLabelV=off  LabelV=Vabc  Vpu=off  VpuLL=off  CurrentMeasurement=yes  SetLabelI=off  LabelI=Iabc  Ipu=off  Pbase=100e6  Vbase=500e3  OutputType=Complex  PhasorSimulation=on  PSBequivalent=0
  dP102_vi : Library/dP102_vi  d=alpha(12)  m=alpha(27)
  dw : Scope
  virtin : powerlib/Elements/Three-Phase Dynamic Load  NominalVoltage=[ 20e3 50 ]  ActiveReactivePowers=[0 0]  PositiveSequence=[1.01728 8.97655]  ExternalControl=on  NpNq="[0  0]"  TimeConstants="[0  0  0  0]"  MinimumVoltage=0.01  Tfilter=1e-1  LoadFlowParameters=[4 50000000 0 0 25000000]
      settings: SourceProductName=Simscape Power Systems  SourceProductBaseCode=PS
  w : Scope
  A : PMIOPort  Port=1  Side=Right
  B : PMIOPort  Port=2  Side=Right
  C : PMIOPort  Port=3  Side=Right
  tag scope: P410=global, Q410=global, w410=global
  wires:
  Mux/1 -> Gain/1
  Gain/1 -> virtin/1
  Constant/1 -> Mux/2
  dP102_vi/1 -> Mux/1
  [Vabc_B410_vi] -> PLL/1
  Mux1/1 -> [w410]
  PLL/1 -> w/1, Mux1/1, dP102_vi/1
  PLL/2 -> dw/1, Mux1/2, dP102_vi/2
  Three-Phase V-I Measurement/1 -> "Power (3ph, Phasor)"/1
  Three-Phase V-I Measurement/2 -> "Power (3ph, Phasor)"/2
  PLL/3 -> Gain1/1
  Gain1/1 -> Mux1/3
  "Power (3ph, Phasor)"/1 -> [P410]
  "Power (3ph, Phasor)"/2 -> [Q410]
  connections:
  Three-Phase V-I Measurement/RConn1 -- A/RConn1
  B/RConn1 -- Three-Phase V-I Measurement/RConn2
  Three-Phase V-I Measurement/RConn3 -- C/RConn1
  virtin/LConn1 -- Three-Phase V-I Measurement/LConn1
  virtin/LConn2 -- Three-Phase V-I Measurement/LConn2
  virtin/LConn3 -- Three-Phase V-I Measurement/LConn3

== system Australian14gen_inertia/VI410_form ==
  Complex to Magnitude-Angle : ComplexToMagnitudeAngle
  Complex to Magnitude-Angle1 : ComplexToMagnitudeAngle
  Demux : Demux  Outputs=[3 3]
  Filter410 : Library/Filter  r=r_fil  l=l_fil  c=c_fil
  Gain : Gain  Gain=[1 0 0]  Multiplication=Matrix(K*u) (u vector)
  Gain1 : Gain  Gain=[1 0 0]  Multiplication=Matrix(K*u) (u vector)
  INV410 : Library/INV  fn=50  Ub=Vbase(12)  Pref=Pinit(12)  ang=thetavsc0(12)  K2=Kvsc(1,12)  K1=Kvsc(2,12)
  Load Flow Bus16 : powerlib/Measurements/Load Flow Bus  Commented=on  LConnTagsString=a  Phases=single  Connectors=on one side  ID=B410_vsw  Vbase=20e3  Vref=1  Vangle=0  VLF=1  VLFb=1  VLFc=1  angleLF=2.825  angleLFb=0  angleLFc=0
      settings: AttributesFormatString=%<ID>\n%<Vbase>V\n%<VLF>pu\n%<angleLF>deg.  SourceProductName=Simscape Power Systems
  Mux : Mux  Inputs=2
  Mux1 : Mux  Inputs=2
  Mux24 : Mux  Inputs=3
  Scope : Scope
  Scope1 : Scope  NumInputPorts=2
  Sum : Sum  Inputs=|+-
  fake_VSC_410 : powerlib/Electrical Sources/Three-Phase Source  Commented=on  InternalConnection=Yg  VoltagePhases=off  Voltage=(20000)*1  PhaseAngle=2.8249  Voltage_phases=[25e3 25e3 25e3]/sqrt(3)  PhaseAngles_phases=[0 -120 +120]  Frequency=50  NonIdealSource=off  SpecifyImpedance=off  Resistance=0  Inductance=0  ShortCircuitLevel=100e6  BaseVoltage=20e3  XRratio=7  BusType=PV  Pref=0  Qref=0  Prefabc=[10e3, 10e3, 10e3]  Qrefabc=[0, 0, 0]  Qmin=-inf  Qmax=inf
  u410 : Constant  Value=0
  A : PMIOPort  Tag=PMCPort  Port=1  Side=Right
  B : PMIOPort  Tag=PMCPort  Port=2  Side=Right
  C : PMIOPort  Tag=PMCPort  Port=3  Side=Right
  tag scope: P410=global, Q410=global, w410=global
  wires:
  u410/1 -> INV410/1
  Filter410/1 -> INV410/2
  INV410/4 -> Mux24/3
  INV410/2 -> Mux24/1
  Filter410/2 -> [Q410]
  INV410/3 -> Mux24/2
  Mux24/1 -> [w410]
  INV410/1 -> [P410]
  Gain1/1 -> Complex to Magnitude-Angle1/1
  Filter410/3 -> Demux/1
  Complex to Magnitude-Angle/1 -> Mux/1
  Mux/1 -> Scope1/1
  Gain/1 -> Complex to Magnitude-Angle/1
  Complex to Magnitude-Angle1/1 -> Mux/2
  Complex to Magnitude-Angle/2 -> Mux1/1
  Mux1/1 -> Scope1/2
  Sum/1 -> Scope/1
  Complex to Magnitude-Angle1/2 -> Mux1/2
  Demux/2 -> Gain1/1, Sum/2
  Demux/1 -> Gain/1, Sum/1
  connections:
  INV410/LConn2 -- fake_VSC_410/RConn2 -- Filter410/LConn2
  Filter410/LConn3 -- Load Flow Bus16/LConn1 -- INV410/LConn3 -- fake_VSC_410/RConn3
  INV410/LConn1 -- Filter410/LConn1 -- fake_VSC_410/RConn1
  Filter410/RConn3 -- C/RConn1
  Filter410/RConn2 -- B/RConn1
  Filter410/RConn1 -- A/RConn1

== system Australian14gen_inertia/VI502 ==
  Constant : Constant  Value=0
  Gain : Gain  Gain=-1
  Gain1 : Gain  Gain=[0 1]  Multiplication=Matrix(K*u) (u vector)
  Mux : Mux  Inputs=2
  Mux1 : Mux  Inputs=3
  PLL : Library/PLL  Kp=PLL_Kp  Ki=PLL_Ki  tau=PLL_tau  theta0=-9.6257  omega0=0
  "Power (3ph, Phasor)" : powerlib_meascontrol/Measurements/Power (3ph, Phasor)
      settings: SourceProductName=Simscape Power Systems  SourceProductBaseCode=PS
  Three-Phase V-I Measurement : powerlib/Measurements/Three-Phase V-I Measurement  VoltageMeasurement=phase-to-ground  SetLabelV=off  LabelV=Vabc  Vpu=off  VpuLL=off  CurrentMeasurement=yes  SetLabelI=off  LabelI=Iabc  Ipu=off  Pbase=100e6  Vbase=500e3  OutputType=Complex  PhasorSimulation=on  PSBequivalent=0
  dP102_vi : Library/dP102_vi  d=alpha(13)  m=alpha(28)
  virtin : powerlib/Elements/Three-Phase Dynamic Load  NominalVoltage=[ 20e3 50 ]  ActiveReactivePowers=[0 0]  PositiveSequence=[0.0544568 -2.58144]  ExternalControl=on  NpNq="[0  0]"  TimeConstants="[0  0  0  0]"  MinimumVoltage=0.01  Tfilter=1e-1  LoadFlowParameters=[4 50000000 0 0 25000000]
      settings: SourceProductName=Simscape Power Systems  SourceProductBaseCode=PS
  A : PMIOPort  Port=1  Side=Right
  B : PMIOPort  Port=2  Side=Right
  C : PMIOPort  Port=3  Side=Right
  tag scope: P502=global, Q502=global, w502=global
  wires:
  Mux/1 -> Gain/1
  Gain/1 -> virtin/1
  Constant/1 -> Mux/2
  dP102_vi/1 -> Mux/1
  [Vabc_B502_vi] -> PLL/1
  PLL/1 -> dP102_vi/1, Mux1/1
  Mux1/1 -> [w502]
  PLL/2 -> Mux1/2, dP102_vi/2
  "Power (3ph, Phasor)"/1 -> [P502]
  Three-Phase V-I Measurement/1 -> "Power (3ph, Phasor)"/1
  "Power (3ph, Phasor)"/2 -> [Q502]
  Three-Phase V-I Measurement/2 -> "Power (3ph, Phasor)"/2
  PLL/3 -> Gain1/1
  Gain1/1 -> Mux1/3
  connections:
  C/RConn1 -- Three-Phase V-I Measurement/RConn3
  B/RConn1 -- Three-Phase V-I Measurement/RConn2
  A/RConn1 -- Three-Phase V-I Measurement/RConn1
  virtin/LConn1 -- Three-Phase V-I Measurement/LConn1
  virtin/LConn2 -- Three-Phase V-I Measurement/LConn2
  Three-Phase V-I Measurement/LConn3 -- virtin/LConn3

== system Australian14gen_inertia/VI502_form ==
  Complex to Magnitude-Angle : ComplexToMagnitudeAngle
  Complex to Magnitude-Angle1 : ComplexToMagnitudeAngle
  Demux : Demux  Outputs=[3 3]
  Filter502 : Library/Filter  r=r_fil  l=l_fil  c=c_fil
  Gain : Gain  Gain=[1 0 0]  Multiplication=Matrix(K*u) (u vector)
  Gain1 : Gain  Gain=[1 0 0]  Multiplication=Matrix(K*u) (u vector)
  INV502 : Library/INV  fn=50  Ub=Vbase(13)  Pref=Pinit(13)  ang=thetavsc0(13)  K2=Kvsc(1,13)  K1=Kvsc(2,13)
  Load Flow Bus18 : powerlib/Measurements/Load Flow Bus  Commented=on  LConnTagsString=a  Phases=single  Connectors=on one side  ID=B502_vsw  Vbase=20e3  Vref=1  Vangle=0  VLF=1  VLFb=1  VLFc=1  angleLF=-12.71  angleLFb=0  angleLFc=0
      settings: AttributesFormatString=%<ID>\n%<Vbase>V\n%<VLF>pu\n%<angleLF>deg.  SourceProductName=Simscape Power Systems
  Mux : Mux  Inputs=2
  Mux1 : Mux  Inputs=2
  Mux22 : Mux  Inputs=3
  Scope : Scope
  Scope1 : Scope  NumInputPorts=2
  Sum : Sum  Inputs=|+-
  fake_VSC_502 : powerlib/Electrical Sources/Three-Phase Source  Commented=on  InternalConnection=Yg  VoltagePhases=off  Voltage=(20000)*1  PhaseAngle=-12.7055  Voltage_phases=[25e3 25e3 25e3]/sqrt(3)  PhaseAngles_phases=[0 -120 +120]  Frequency=50  NonIdealSource=off  SpecifyImpedance=off  Resistance=0  Inductance=0  ShortCircuitLevel=100e6  BaseVoltage=20e3  XRratio=7  BusType=PV  Pref=0  Qref=0  Prefabc=[10e3, 10e3, 10e3]  Qrefabc=[0, 0, 0]  Qmin=-inf  Qmax=inf
  u502 : Constant  Value=0
  A : PMIOPort  Port=1  Side=Left
  B : PMIOPort  Port=2  Side=Left
  C : PMIOPort  Port=3  Side=Left
  tag scope: P502=global, Q502=global, w502=global
  wires:
  u502/1 -> INV502/1
  Filter502/1 -> INV502/2
  Filter502/2 -> [Q502]
  Mux22/1 -> [w502]
  INV502/2 -> Mux22/1
  INV502/3 -> Mux22/2
  INV502/4 -> Mux22/3
  INV502/1 -> [P502]
  Mux/1 -> Scope1/1
  Sum/1 -> Scope/1
  Complex to Magnitude-Angle1/2 -> Mux1/2
  Gain/1 -> Complex to Magnitude-Angle/1
  Complex to Magnitude-Angle/1 -> Mux/1
  Demux/2 -> Gain1/1, Sum/2
  Filter502/3 -> Demux/1
  Demux/1 -> Gain/1, Sum/1
  Complex to Magnitude-Angle/2 -> Mux1/1
  Gain1/1 -> Complex to Magnitude-Angle1/1
  Mux1/1 -> Scope1/2
  Complex to Magnitude-Angle1/1 -> Mux/2
  connections:
  INV502/LConn3 -- Load Flow Bus18/LConn1 -- Filter502/LConn3 -- fake_VSC_502/RConn3
  INV502/LConn1 -- fake_VSC_502/RConn1 -- Filter502/LConn1
  INV502/LConn2 -- fake_VSC_502/RConn2 -- Filter502/LConn2
  C/RConn1 -- Filter502/RConn3
  B/RConn1 -- Filter502/RConn2
  A/RConn1 -- Filter502/RConn1

== system Australian14gen_inertia/VI504 ==
  Constant : Constant  Value=0
  Gain : Gain  Gain=-1
  Gain1 : Gain  Gain=[0 1]  Multiplication=Matrix(K*u) (u vector)
  Mux : Mux  Inputs=2
  Mux1 : Mux  Inputs=3
  PLL : Library/PLL  Kp=PLL_Kp  Ki=PLL_Ki  tau=PLL_tau  theta0=-12.1555  omega0=0
  "Power (3ph, Phasor)" : powerlib_meascontrol/Measurements/Power (3ph, Phasor)
      settings: SourceProductName=Simscape Power Systems  SourceProductBaseCode=PS
  Three-Phase V-I Measurement : powerlib/Measurements/Three-Phase V-I Measurement  VoltageMeasurement=phase-to-ground  SetLabelV=off  LabelV=Vabc  Vpu=off  VpuLL=off  CurrentMeasurement=yes  SetLabelI=off  LabelI=Iabc  Ipu=off  Pbase=100e6  Vbase=500e3  OutputType=Complex  PhasorSimulation=on  PSBequivalent=0
  dP102_vi : Library/dP102_vi  d=alpha(14)  m=alpha(29)
  virtin : powerlib/Elements/Three-Phase Dynamic Load  NominalVoltage=[ 20e3 50 ]  ActiveReactivePowers=[0 0]  PositiveSequence=[1.03954 -12.1555]  ExternalControl=on  NpNq="[0  0]"  TimeConstants="[0  0  0  0]"  MinimumVoltage=0.01  Tfilter=1e-1  LoadFlowParameters=[4 50000000 0 0 25000000]
      settings: SourceProductName=Simscape Power Systems  SourceProductBaseCode=PS
  A : PMIOPort  Port=1  Side=Right
  B : PMIOPort  Port=2  Side=Right
  C : PMIOPort  Port=3  Side=Right
  tag scope: P504=global, Q504=global, w504=global
  wires:
  Mux/1 -> Gain/1
  Gain/1 -> virtin/1
  Constant/1 -> Mux/2
  dP102_vi/1 -> Mux/1
  [Vabc_B504_vi] -> PLL/1
  PLL/1 -> Mux1/1, dP102_vi/1
  Mux1/1 -> [w504]
  PLL/2 -> Mux1/2, dP102_vi/2
  "Power (3ph, Phasor)"/1 -> [P504]
  Three-Phase V-I Measurement/1 -> "Power (3ph, Phasor)"/1
  "Power (3ph, Phasor)"/2 -> [Q504]
  Three-Phase V-I Measurement/2 -> "Power (3ph, Phasor)"/2
  PLL/3 -> Gain1/1
  Gain1/1 -> Mux1/3
  connections:
  C/RConn1 -- Three-Phase V-I Measurement/RConn3
  B/RConn1 -- Three-Phase V-I Measurement/RConn2
  A/RConn1 -- Three-Phase V-I Measurement/RConn1
  virtin/LConn3 -- Three-Phase V-I Measurement/LConn3
  virtin/LConn2 -- Three-Phase V-I Measurement/LConn2
  virtin/LConn1 -- Three-Phase V-I Measurement/LConn1
